simulink model "project_simulink"  (R2025b)
settings: Solver=FixedStepAuto  StartTime=0.0  StopTime=inf  FixedStep=0.005  RelTol=1e-3
undefined symbols (not defined in the file or in its folder): NULL
libraries: dspstat3 x3, instrumentseriallib x2
settings Model: Creator=ateeq  LastModifiedBy=ateeq

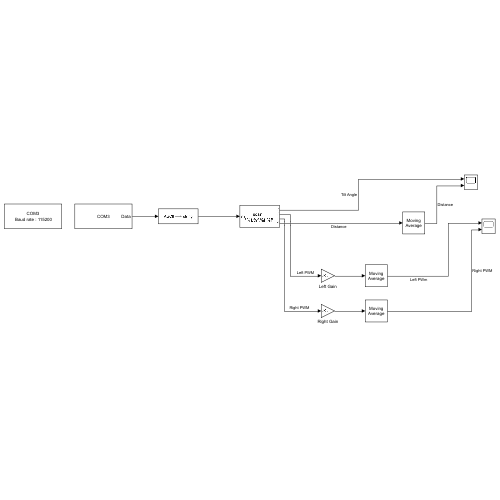
[thumbnail: Simulink's stored preview of the top-level diagram]
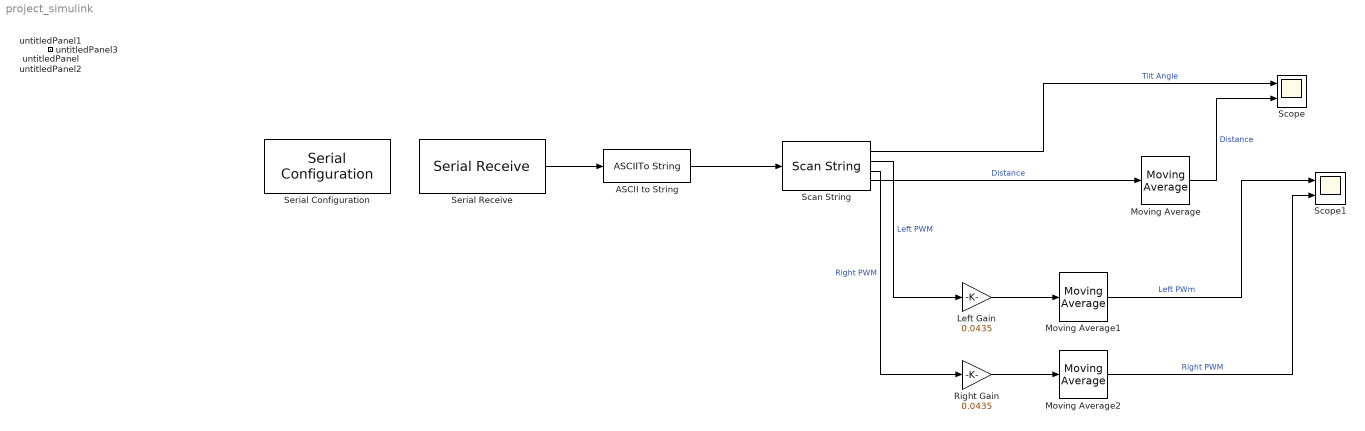
== system project_simulink ==
  ASCII to String : ASCIIToString
  Left Gain : Gain  Gain=0.0435
  Moving Average : dspstat3/Moving Average  Method=Sliding window  ForgettingFactorPort=off  SpecifyWindowLength=on  WindowLength=20  OverlapLength=3  AllowArbitraryInputLength=on  ForgettingFactor=0.9  SimulateUsing=Interpreted execution
  Moving Average1 : dspstat3/Moving Average  Method=Sliding window  ForgettingFactorPort=off  SpecifyWindowLength=on  WindowLength=5  OverlapLength=3  AllowArbitraryInputLength=on  ForgettingFactor=0.9  SimulateUsing=Interpreted execution
  Moving Average2 : dspstat3/Moving Average  Method=Sliding window  ForgettingFactorPort=off  SpecifyWindowLength=on  WindowLength=5  OverlapLength=3  AllowArbitraryInputLength=on  ForgettingFactor=0.9  SimulateUsing=Interpreted execution
  Right Gain : Gain  Gain=0.0435
  Scan String : ScanString  Format="\"%f,%f,%f,%f\""
  Scope : Scope  NumInputPorts=2
      settings: ActiveDisplayYMinimum=-1  ActiveDisplayYMaximum=1
  Scope1 : Scope  NumInputPorts=2
      settings: ActiveDisplayYMinimum=-4933.6411743164062  ActiveDisplayYMaximum=4828.4712524414062
  Serial Configuration : instrumentseriallib/Serial Configuration  Priority=-200000  PortSel=COM3  Port=COM3  ComPort=COM3  BaudRate=115200  DataBits=8  Parity=none  StopBits=1  ByteOrder=little-endian  FlowControl=none  Timeout=10  SimulateUsing=Interpreted execution  BlockInModel=on  aMode=1
  Serial Receive : instrumentseriallib/Serial Receive  Priority=1  PortSel=COM3  Port=COM3  ComPort=COM3  DataType=uint8  SaveDataType=uint8  ToggleHeader=off  Header=[]  ToggleDataSize=on  DataSize=[64 1]  ToggleTerminator=on  Terminator=NULL ('\0')  CustomTerminator=10  InputFormat=Column major  EnableBlockingMode=on  ActionDataUnavailable=Output last received value  ActionWhenDataUnavailable=Output last received value  CustomValue=0  SampleTime=0.005  SimulateUsing=Interpreted execution  BlockInModel=on  aMode=1  LibraryInUse=instrumentlib
  untitledPanel : Subsystem  Tag=HiddenForWebPanel  IsWebBlockPanel=on
  untitledPanel1 : Subsystem  Tag=HiddenForWebPanel  IsWebBlockPanel=on
  untitledPanel2 : Subsystem  Tag=HiddenForWebPanel  IsWebBlockPanel=on
  untitledPanel3 : Subsystem  Tag=HiddenForWebPanel  IsWebBlockPanel=on
  wires:
  Serial Receive/1 -> ASCII to String/1
  ASCII to String/1 -> Scan String/1
  Scan String/2 -> Left Gain/1  "Left PWM"
  Scan String/3 -> Right Gain/1  "Right PWM"
  Scan String/4 -> Moving Average/1  "Distance"
  Left Gain/1 -> Moving Average1/1
  Right Gain/1 -> Moving Average2/1
  Moving Average2/1 -> Scope1/2  "Right PWM"
  Moving Average1/1 -> Scope1/1  "Left PWm"
  Moving Average/1 -> Scope/2  "Distance"
  Scan String/1 -> Scope/1  "Tilt Angle"

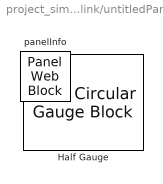
== system project_simulink/untitledPanel ==
  Half Gauge : SemiCircularGaugeBlock  Tag=HiddenForWebPanel  PanelInfo="{\"height\":96,\"left\":18,\"panelId\":\"panelId-6f800675-98d9-4a9f-ad54-afe5ae169253\",\"top\":18,\"type\":\"panelChild\",\"version\":\"2019b\",\"width\":120,\"zIndex\":1500002}"  ScaleMin=-12  ScaleMax=12  FontColor=[0.0, 0.0, 0.0]
  panelInfo : PanelWebBlock  Tag=HiddenForWebPanel  PanelInfo="{\"compacted\":false,\"height\":136,\"isActiveTab\":true,\"left\":1256,\"name\":\"Panel\",\"panelId\":\"panelId-6f800675-98d9-4a9f-ad54-afe5ae169253\",\"tabIndex\":0,\"tabbedSetId\":\"tabbedSet3506691936\",\"top\":340,\"type\":\"panel\",\"version\":\"2019b\",\"visible\":true,\"width\":160,\"zIndex\":1500002}"

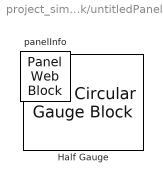
== system project_simulink/untitledPanel1 ==
  Half Gauge : SemiCircularGaugeBlock  Tag=HiddenForWebPanel  PanelInfo="{\"height\":96,\"left\":18,\"panelId\":\"panelId-2e0b96b9-fde5-485d-8c46-e10fb5141348\",\"top\":18,\"type\":\"panelChild\",\"version\":\"2019b\",\"width\":120,\"zIndex\":1500002}"  ScaleMin=-12  ScaleMax=12  FontColor=[0.0, 0.0, 0.0]
  panelInfo : PanelWebBlock  Tag=HiddenForWebPanel  PanelInfo="{\"compacted\":false,\"height\":136,\"isActiveTab\":true,\"left\":1255,\"name\":\"Panel1\",\"panelId\":\"panelId-2e0b96b9-fde5-485d-8c46-e10fb5141348\",\"tabIndex\":0,\"tabbedSetId\":\"tabbedSet4856572872\",\"top\":174,\"type\":\"panel\",\"version\":\"2019b\",\"visible\":true,\"width\":160,\"zIndex\":1500004}"

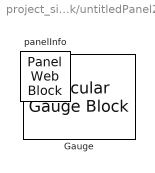
== system project_simulink/untitledPanel2 ==
  Gauge : CircularGaugeBlock  Tag=HiddenForWebPanel  PanelInfo="{\"height\":85,\"left\":18,\"panelId\":\"panelId-2eaf436e-4f06-47f3-b669-1f04f0b1e40f\",\"top\":18,\"type\":\"panelChild\",\"version\":\"2019b\",\"width\":112,\"zIndex\":1500002}"  ScaleMin=-45  ScaleMax=45  FontColor=[0.0, 0.0, 0.0]
  panelInfo : PanelWebBlock  Tag=HiddenForWebPanel  PanelInfo="{\"compacted\":false,\"height\":125,\"isActiveTab\":true,\"left\":1256,\"name\":\"Panel2\",\"panelId\":\"panelId-2eaf436e-4f06-47f3-b669-1f04f0b1e40f\",\"tabIndex\":0,\"tabbedSetId\":\"tabbedSet9039577401\",\"top\":32,\"type\":\"panel\",\"version\":\"2019b\",\"visible\":true,\"width\":152,\"zIndex\":1500006}"

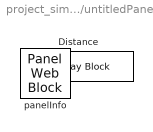
== system project_simulink/untitledPanel3 ==
  Distance : DisplayBlock  Tag=HiddenForWebPanel  PanelInfo="{\"height\":30,\"left\":18,\"panelId\":\"panelId-60362c40-2027-4038-8fd2-8c7509474957\",\"top\":18,\"type\":\"panelChild\",\"version\":\"2019b\",\"width\":110,\"zIndex\":1500002}"  LabelPosition=Hide  Transparency=1  GridColor=[0.502, 0.502, 0.502]
  panelInfo : PanelWebBlock  Tag=HiddenForWebPanel  PanelInfo="{\"compacted\":false,\"height\":70,\"isActiveTab\":true,\"left\":1081,\"name\":\"Panel3\",\"panelId\":\"panelId-60362c40-2027-4038-8fd2-8c7509474957\",\"tabIndex\":0,\"tabbedSetId\":\"tabbedSet6524163499\",\"top\":452,\"type\":\"panel\",\"version\":\"2019b\",\"visible\":true,\"width\":150,\"zIndex\":1500008}"  PanelSnapshot=<binary blob, 6368 chars, not shown>
